simulink library "AtomicLibrary"
PostLoadFcn:
  | PacketBusGenerator; RailCabBusGenerator
(part 6 of 8)

== matlab function UserInterface/Link Layer HMI_STRATEGYREQUEST.provider/Receive Packet ==
  data: packetFrom input; packetMsg input; packetParam input; eventQueueIn input uint8; eventParamQueueIn input double; eventQueue output uint8; eventParamQueue output double; bufferOverflow output boolean
function [eventQueue, eventParamQueue, bufferOverflow] = receivePacket(packetFrom, packetMsg, packetParam, eventQueueIn, eventParamQueueIn)
%#eml
% This function receives packets and adds them to the event queue.
% A packet consists of a source, a message and an optional parameter for 
% the message. Source and message are contained at position 1 and 2 in the 
% eventQueue. Because of the different data type the parameter has his own 
% queue eventParamQueue.

%Constants
SOURCE = 2;
MESSAGE = 1;
BUS_SIZE = numel(packetFrom);
QUEUE_SIZE = 10;

%Init
eventQueue = eventQueueIn;
eventParamQueue = eventParamQueueIn;
bufferOverflow = false;

%New incoming packet
for i = 1:BUS_SIZE
    if packetFrom(i) ~= 0 
        bufferOverflow = true;
        %Add it to the incoming event Queue
        for j = 1:QUEUE_SIZE
            %Search for an empty place
            if eventQueue(j,SOURCE) == 0
                eventQueue(j,SOURCE)    = packetFrom(i);
                eventQueue(j,MESSAGE)   = packetMsg(i);
                eventParamQueue(j)      = packetParam(i);
                bufferOverflow = false;
                break;
            end
        end        
    else
        break;
    end
end

== matlab function UserInterface/Link Layer HMI_STRATEGYREQUEST.provider/Send Packet ==
  data: busSizeSignal input; eventQueueIn input uint8; eventParamQueueIn input double; packetMsg output; packetParam output; eventQueue output uint8; eventParamQueue output double
function [packetMsg, packetParam, eventQueue, eventParamQueue] = sendPacket(busSizeSignal, eventQueueIn, eventParamQueueIn)
%#eml

% This function creates packets from the event queue. A packet consists
% of a destination, a message and an optional parameter for the message.
% Destination and message are contained at position 1 and 2 in the 
% eventQueue. Because of the different data type the parameter has his own 
% queue eventParamQueue.

%Constants
DESTINATION = 2;
MESSAGE = 1;
QUEUE_SIZE = 10;

busSize = numel(busSizeSignal);

%Init
eventQueue = eventQueueIn;
eventParamQueue = eventParamQueueIn;
packetMsg = zeros(1,busSize,'uint16');
packetParam = zeros(1,busSize,'double');

%There is an event in the queue
for i = 1:busSize   
    if eventQueue(1,DESTINATION) ~= 0 || eventQueue(1,MESSAGE) ~= 0
        %Create packet from the firs entry in the queue
        packetMsg(i)   = uint16(eventQueue(1,MESSAGE));
        packetParam(i) = eventParamQueue(1);
        %Remove the event from the queue
        for j=1:QUEUE_SIZE - 1
            eventQueue(j,DESTINATION)   = eventQueue(j+1,DESTINATION);
            eventQueue(j,MESSAGE)       = eventQueue(j+1,MESSAGE);
            eventParamQueue(j)          = eventParamQueue(j+1);
        end
        %Set last element to zero
        eventQueue(QUEUE_SIZE,DESTINATION)  = 0;
        eventQueue(QUEUE_SIZE,MESSAGE)      = 0;
        eventParamQueue(QUEUE_SIZE)    = 0;
    else
        break;
    end
end

== matlab function UserInterface/Link Layer HMI_RESET.master/DataLinkLayer/Embedded MATLAB Function ==
  data: snd_from_in input; snd_to_in input; snd_msg_in input; snd_param_in input; recv_from_in input; recv_to_in input; recv_msg_in input; recv_param_in input; recv_pkgid_in input uint32; recv_time_in input; currentTime input; from output; to output; msg output; param output; pkgid output; recv_from_out output; recv_msg_out output; recv_param_out output; time output; queue_sending_ratio output; queue_received_ratio output; queue_ack_ratio output
function [from, to, msg, param, pkgid, recv_from_out, recv_msg_out, recv_param_out, time, queue_sending_ratio, queue_received_ratio, queue_ack_ratio] = ackHandler(snd_from_in, snd_to_in, snd_msg_in, snd_param_in, recv_from_in, recv_to_in, recv_msg_in, recv_param_in, recv_pkgid_in, recv_time_in, currentTime)
%#eml
eml.extrinsic('warning', 'disp', 'fprintf');

%Constants
BUS_SIZE =  numel(snd_msg_in);
TIMEOUT_ACK     = 2.0;
MSG_ACK         = 255;
QUEUE_SIZE_SENDING = 10 * BUS_SIZE;
QUEUE_SIZE_ACK  = 10* BUS_SIZE;
QUEUE_SIZE_RECEIVED = 10 *BUS_SIZE;


%Init
from    = zeros(1,BUS_SIZE,'uint8');
to      = zeros(1,BUS_SIZE,'uint8');
msg     = zeros(1,BUS_SIZE,'uint16');
param   = zeros(1,BUS_SIZE,'double');
pkgid   = zeros(1,BUS_SIZE,'uint32');
time    = zeros(1,BUS_SIZE,'double');
 
recv_from_out    = zeros(1,BUS_SIZE,'uint8');
recv_msg_out     = zeros(1,BUS_SIZE,'uint16');
recv_param_out   = zeros(1,BUS_SIZE,'double');


recv_in = bus(recv_from_in, recv_to_in, recv_msg_in, recv_param_in, recv_pkgid_in, recv_time_in, BUS_SIZE);



%Persistent variables
persistent sendingQueue ackQueue receivedQueue lastPkgid

if isempty(lastPkgid)
    lastPkgid = uint32(0);
end

if isempty(sendingQueue)
    sendingQueue = repmat(packet(0,0,0,0,0,0), 1, QUEUE_SIZE_SENDING);
end

if isempty(ackQueue)
    ackQueue = repmat(packet(0,0,0,0,0,0), 1, QUEUE_SIZE_ACK);
end

if isempty(receivedQueue)
    receivedQueue = repmat(packet(0, 0, 0, 0, 0, 0), 1, QUEUE_SIZE_RECEIVED);
end

%compute stats
queue_sending_ratio = queueNumElements(sendingQueue)/QUEUE_SIZE_SENDING;
queue_ack_ratio = queueNumElements(ackQueue)/QUEUE_SIZE_ACK;
queue_received_ratio = queueNumElements(receivedQueue)/QUEUE_SIZE_RECEIVED;

%Step 1: Check for a new outgoing packet
for i = 1:BUS_SIZE    
    if snd_msg_in(i) ~= 0
        lastPkgid = lastPkgid +1;
        outgoing = packet(snd_from_in, snd_to_in, snd_msg_in(i), snd_param_in(i), lastPkgid, currentTime);

        %Add packet so the outgoing queue
        sendingQueue = enqueue(sendingQueue, outgoing); 
    end
end
    
%Step 2: Check for a new incoming packet
for i = 1:length(recv_in)
    incoming = packet(recv_in(i).from, recv_in(i).to, recv_in(i).msg, recv_in(i).param, recv_in(i).pkgid, recv_in(i).time);
    if incoming.from ~= 0 && incoming.to == snd_from_in
        if incoming.msg == MSG_ACK
            %Remove packet from ackQueue
            for j=1:length(ackQueue)
                if ackQueue(j).pkgid == uint32(incoming.param)
                    ackQueue = dequeue(ackQueue,j);
                    break;
                end
            end
        else
            %Send ACK
            ackPacket = packet(incoming.to, incoming.from, MSG_ACK, double(incoming.pkgid),incoming.pkgid, currentTime);
            sendingQueue = enqueue(sendingQueue,ackPacket);

            %Check for duplicated packets
            duplicatedPacket = false;
            for j=1:length(receivedQueue)
                if receivedQueue(j).pkgid == incoming.pkgid && receivedQueue(j).from == incoming.from
                    duplicatedPacket = true;
                    break;
                end
            end

            if duplicatedPacket == false
                %save packet
                receivedQueue = enqueue(receivedQueue, incoming);            
            end
        end
    end
end

%Step 3: Forward incoming packet
for i = 1:BUS_SIZE
    if receivedQueue(1).from ~= 0
        recv_from_out(i)    = receivedQueue(1).from;
        recv_msg_out(i)     = receivedQueue(1).msg;
        recv_param_out(i)   = receivedQueue(1).param;
        receivedQueue = dequeue(receivedQueue,1);
    else
        break;
    end
end

%Step 4: Timeout reached? Send packet again
for i = 1:length(ackQueue)
    if ackQueue(i).to ~= 0
        if ackQueue(i).time + TIMEOUT_ACK <= currentTime
            %Reset counter
            ackQueue(i).time = currentTime;
            %Send again
            sendingQueue = enqueue(sendingQueue, ackQueue(i));
            %Remove packet from ackQueue
            ackQueue = dequeue(ackQueue, i);
        end
    end
end


%Step 5: Send outgoing packet
for i = 1:BUS_SIZE
    if sendingQueue(1).to ~= 0    
        from(i)    = sendingQueue(1).from;
        to(i)      = sendingQueue(1).to;
        msg(i)     = sendingQueue(1).msg;
        param(i)   = sendingQueue(1).param;
        pkgid(i)   = sendingQueue(1).pkgid;
        time(i)    = sendingQueue(1).time;

        %Add it to the ack queue
        if sendingQueue(1).msg ~= MSG_ACK
            ackQueue = enqueue(ackQueue, sendingQueue(1));
        end

        %remove packet from sending queue
        sendingQueue = dequeue(sendingQueue, 1);    
    else
        break;
    end
end


%%%%%%%%%%%%%%%%%%%%%%%%%%%%%%%%%%%%%%%%%%%%%%%%%%%%%%%%%%%%%%%%%%%%%%%%%%%
%%                          H E L P E R
%%%%%%%%%%%%%%%%%%%%%%%%%%%%%%%%%%%%%%%%%%%%%%%%%%%%%%%%%%%%%%%%%%%%%%%%%%%

function p = packet(from, to, msg, param, pkgid, time)
%#eml
%Defines a packet
p = struct('from', uint8(from),'to', uint8(to),'msg', uint16(msg),'param', double(param),'pkgid', uint32(pkgid), 'time', double(time));

function bus = bus(from, to, msg, param, pkgid, time, size) %emp
%Create an empty bus
bus = repmat(packet(0,0,0,0,0,0), 1, size);
for i=1:size
    bus(i) = packet(from(i), to(i), msg(i), param(i), pkgid(i), time(i));
end


function queue = enqueue(queue, packet)
%#eml
eml.extrinsic('warning', 'sprintf');
for i = 1:length(queue)
    if queue(i).to == 0
        queue(i) = packet;
        return;
    end
end
warning('RailCab:DataLinkLayer', 'DataLinkLayer Buffer overflow. Dropping packet  %3u: %u->%u :%3u (%.1f) @%.2f', packet.pkgid, packet.from, packet.to, packet.msg, packet.param, packet.time);

function queue = dequeue(queue, index)
%#eml
assert(index <= length(queue))
for i=index:length(queue)-1;
    queue(i) = queue(i+1);
end
queue(length(queue)) = packet(0,0,0,0,0,0);

function num = queueNumElements(queue)
%#eml
num = 0;
for i = 1:length(queue)
    if queue(i).to ~= uint8(0)
        num = num+1;
    end
end    

function packetString = toString(packet) %#eml
eml.extrinsic('sprintf');
packetString = sprintf('%3u: %u->%u :%3u (%.1f) @%.2f', packet.pkgid, packet.from, packet.to, packet.msg, packet.param, packet.time);

== matlab function UserInterface/Link Layer HMI_RESET.master/Receive Packet ==
  data: packetFrom input; packetMsg input; packetParam input; eventQueueIn input uint8; eventParamQueueIn input double; eventQueue output uint8; eventParamQueue output double; bufferOverflow output boolean
function [eventQueue, eventParamQueue, bufferOverflow] = receivePacket(packetFrom, packetMsg, packetParam, eventQueueIn, eventParamQueueIn)
%#eml
% This function receives packets and adds them to the event queue.
% A packet consists of a source, a message and an optional parameter for 
% the message. Source and message are contained at position 1 and 2 in the 
% eventQueue. Because of the different data type the parameter has his own 
% queue eventParamQueue.

%Constants
SOURCE = 2;
MESSAGE = 1;
BUS_SIZE = numel(packetFrom);
QUEUE_SIZE = 10;

%Init
eventQueue = eventQueueIn;
eventParamQueue = eventParamQueueIn;
bufferOverflow = false;

%New incoming packet
for i = 1:BUS_SIZE
    if packetFrom(i) ~= 0 
        bufferOverflow = true;
        %Add it to the incoming event Queue
        for j = 1:QUEUE_SIZE
            %Search for an empty place
            if eventQueue(j,SOURCE) == 0
                eventQueue(j,SOURCE)    = packetFrom(i);
                eventQueue(j,MESSAGE)   = packetMsg(i);
                eventParamQueue(j)      = packetParam(i);
                bufferOverflow = false;
                break;
            end
        end        
    else
        break;
    end
end

== matlab function UserInterface/Link Layer HMI_RESET.master/Send Packet ==
  data: busSizeSignal input; eventQueueIn input uint8; eventParamQueueIn input double; packetMsg output; packetParam output; eventQueue output uint8; eventParamQueue output double
function [packetMsg, packetParam, eventQueue, eventParamQueue] = sendPacket(busSizeSignal, eventQueueIn, eventParamQueueIn)
%#eml

% This function creates packets from the event queue. A packet consists
% of a destination, a message and an optional parameter for the message.
% Destination and message are contained at position 1 and 2 in the 
% eventQueue. Because of the different data type the parameter has his own 
% queue eventParamQueue.

%Constants
DESTINATION = 2;
MESSAGE = 1;
QUEUE_SIZE = 10;

busSize = numel(busSizeSignal);

%Init
eventQueue = eventQueueIn;
eventParamQueue = eventParamQueueIn;
packetMsg = zeros(1,busSize,'uint16');
packetParam = zeros(1,busSize,'double');

%There is an event in the queue
for i = 1:busSize   
    if eventQueue(1,DESTINATION) ~= 0 || eventQueue(1,MESSAGE) ~= 0
        %Create packet from the firs entry in the queue
        packetMsg(i)   = uint16(eventQueue(1,MESSAGE));
        packetParam(i) = eventParamQueue(1);
        %Remove the event from the queue
        for j=1:QUEUE_SIZE - 1
            eventQueue(j,DESTINATION)   = eventQueue(j+1,DESTINATION);
            eventQueue(j,MESSAGE)       = eventQueue(j+1,MESSAGE);
            eventParamQueue(j)          = eventParamQueue(j+1);
        end
        %Set last element to zero
        eventQueue(QUEUE_SIZE,DESTINATION)  = 0;
        eventQueue(QUEUE_SIZE,MESSAGE)      = 0;
        eventParamQueue(QUEUE_SIZE)    = 0;
    else
        break;
    end
end

== matlab function UserInterface/Link Layer HMI_STRATEGY.master/DataLinkLayer/Embedded MATLAB Function ==
  data: snd_from_in input; snd_to_in input; snd_msg_in input; snd_param_in input; recv_from_in input; recv_to_in input; recv_msg_in input; recv_param_in input; recv_pkgid_in input uint32; recv_time_in input; currentTime input; from output; to output; msg output; param output; pkgid output; recv_from_out output; recv_msg_out output; recv_param_out output; time output; queue_sending_ratio output; queue_received_ratio output; queue_ack_ratio output
function [from, to, msg, param, pkgid, recv_from_out, recv_msg_out, recv_param_out, time, queue_sending_ratio, queue_received_ratio, queue_ack_ratio] = ackHandler(snd_from_in, snd_to_in, snd_msg_in, snd_param_in, recv_from_in, recv_to_in, recv_msg_in, recv_param_in, recv_pkgid_in, recv_time_in, currentTime)
%#eml
eml.extrinsic('warning', 'disp', 'fprintf');

%Constants
BUS_SIZE =  numel(snd_msg_in);
TIMEOUT_ACK     = 2.0;
MSG_ACK         = 255;
QUEUE_SIZE_SENDING = 10 * BUS_SIZE;
QUEUE_SIZE_ACK  = 10* BUS_SIZE;
QUEUE_SIZE_RECEIVED = 10 *BUS_SIZE;


%Init
from    = zeros(1,BUS_SIZE,'uint8');
to      = zeros(1,BUS_SIZE,'uint8');
msg     = zeros(1,BUS_SIZE,'uint16');
param   = zeros(1,BUS_SIZE,'double');
pkgid   = zeros(1,BUS_SIZE,'uint32');
time    = zeros(1,BUS_SIZE,'double');
 
recv_from_out    = zeros(1,BUS_SIZE,'uint8');
recv_msg_out     = zeros(1,BUS_SIZE,'uint16');
recv_param_out   = zeros(1,BUS_SIZE,'double');


recv_in = bus(recv_from_in, recv_to_in, recv_msg_in, recv_param_in, recv_pkgid_in, recv_time_in, BUS_SIZE);



%Persistent variables
persistent sendingQueue ackQueue receivedQueue lastPkgid

if isempty(lastPkgid)
    lastPkgid = uint32(0);
end

if isempty(sendingQueue)
    sendingQueue = repmat(packet(0,0,0,0,0,0), 1, QUEUE_SIZE_SENDING);
end

if isempty(ackQueue)
    ackQueue = repmat(packet(0,0,0,0,0,0), 1, QUEUE_SIZE_ACK);
end

if isempty(receivedQueue)
    receivedQueue = repmat(packet(0, 0, 0, 0, 0, 0), 1, QUEUE_SIZE_RECEIVED);
end

%compute stats
queue_sending_ratio = queueNumElements(sendingQueue)/QUEUE_SIZE_SENDING;
queue_ack_ratio = queueNumElements(ackQueue)/QUEUE_SIZE_ACK;
queue_received_ratio = queueNumElements(receivedQueue)/QUEUE_SIZE_RECEIVED;

%Step 1: Check for a new outgoing packet
for i = 1:BUS_SIZE    
    if snd_msg_in(i) ~= 0
        lastPkgid = lastPkgid +1;
        outgoing = packet(snd_from_in, snd_to_in, snd_msg_in(i), snd_param_in(i), lastPkgid, currentTime);

        %Add packet so the outgoing queue
        sendingQueue = enqueue(sendingQueue, outgoing); 
    end
end
    
%Step 2: Check for a new incoming packet
for i = 1:length(recv_in)
    incoming = packet(recv_in(i).from, recv_in(i).to, recv_in(i).msg, recv_in(i).param, recv_in(i).pkgid, recv_in(i).time);
    if incoming.from ~= 0 && incoming.to == snd_from_in
        if incoming.msg == MSG_ACK
            %Remove packet from ackQueue
            for j=1:length(ackQueue)
                if ackQueue(j).pkgid == uint32(incoming.param)
                    ackQueue = dequeue(ackQueue,j);
                    break;
                end
            end
        else
            %Send ACK
            ackPacket = packet(incoming.to, incoming.from, MSG_ACK, double(incoming.pkgid),incoming.pkgid, currentTime);
            sendingQueue = enqueue(sendingQueue,ackPacket);

            %Check for duplicated packets
            duplicatedPacket = false;
            for j=1:length(receivedQueue)
                if receivedQueue(j).pkgid == incoming.pkgid && receivedQueue(j).from == incoming.from
                    duplicatedPacket = true;
                    break;
                end
            end

            if duplicatedPacket == false
                %save packet
                receivedQueue = enqueue(receivedQueue, incoming);            
            end
        end
    end
end

%Step 3: Forward incoming packet
for i = 1:BUS_SIZE
    if receivedQueue(1).from ~= 0
        recv_from_out(i)    = receivedQueue(1).from;
        recv_msg_out(i)     = receivedQueue(1).msg;
        recv_param_out(i)   = receivedQueue(1).param;
        receivedQueue = dequeue(receivedQueue,1);
    else
        break;
    end
end

%Step 4: Timeout reached? Send packet again
for i = 1:length(ackQueue)
    if ackQueue(i).to ~= 0
        if ackQueue(i).time + TIMEOUT_ACK <= currentTime
            %Reset counter
            ackQueue(i).time = currentTime;
            %Send again
            sendingQueue = enqueue(sendingQueue, ackQueue(i));
            %Remove packet from ackQueue
            ackQueue = dequeue(ackQueue, i);
        end
    end
end


%Step 5: Send outgoing packet
for i = 1:BUS_SIZE
    if sendingQueue(1).to ~= 0    
        from(i)    = sendingQueue(1).from;
        to(i)      = sendingQueue(1).to;
        msg(i)     = sendingQueue(1).msg;
        param(i)   = sendingQueue(1).param;
        pkgid(i)   = sendingQueue(1).pkgid;
        time(i)    = sendingQueue(1).time;

        %Add it to the ack queue
        if sendingQueue(1).msg ~= MSG_ACK
            ackQueue = enqueue(ackQueue, sendingQueue(1));
        end

        %remove packet from sending queue
        sendingQueue = dequeue(sendingQueue, 1);    
    else
        break;
    end
end


%%%%%%%%%%%%%%%%%%%%%%%%%%%%%%%%%%%%%%%%%%%%%%%%%%%%%%%%%%%%%%%%%%%%%%%%%%%
%%                          H E L P E R
%%%%%%%%%%%%%%%%%%%%%%%%%%%%%%%%%%%%%%%%%%%%%%%%%%%%%%%%%%%%%%%%%%%%%%%%%%%

function p = packet(from, to, msg, param, pkgid, time)
%#eml
%Defines a packet
p = struct('from', uint8(from),'to', uint8(to),'msg', uint16(msg),'param', double(param),'pkgid', uint32(pkgid), 'time', double(time));

function bus = bus(from, to, msg, param, pkgid, time, size) %emp
%Create an empty bus
bus = repmat(packet(0,0,0,0,0,0), 1, size);
for i=1:size
    bus(i) = packet(from(i), to(i), msg(i), param(i), pkgid(i), time(i));
end


function queue = enqueue(queue, packet)
%#eml
eml.extrinsic('warning', 'sprintf');
for i = 1:length(queue)
    if queue(i).to == 0
        queue(i) = packet;
        return;
    end
end
warning('RailCab:DataLinkLayer', 'DataLinkLayer Buffer overflow. Dropping packet  %3u: %u->%u :%3u (%.1f) @%.2f', packet.pkgid, packet.from, packet.to, packet.msg, packet.param, packet.time);

function queue = dequeue(queue, index)
%#eml
assert(index <= length(queue))
for i=index:length(queue)-1;
    queue(i) = queue(i+1);
end
queue(length(queue)) = packet(0,0,0,0,0,0);

function num = queueNumElements(queue)
%#eml
num = 0;
for i = 1:length(queue)
    if queue(i).to ~= uint8(0)
        num = num+1;
    end
end    

function packetString = toString(packet) %#eml
eml.extrinsic('sprintf');
packetString = sprintf('%3u: %u->%u :%3u (%.1f) @%.2f', packet.pkgid, packet.from, packet.to, packet.msg, packet.param, packet.time);

== matlab function UserInterface/Link Layer HMI_STRATEGY.master/Receive Packet ==
  data: packetFrom input; packetMsg input; packetParam input; eventQueueIn input uint8; eventParamQueueIn input double; eventQueue output uint8; eventParamQueue output double; bufferOverflow output boolean
function [eventQueue, eventParamQueue, bufferOverflow] = receivePacket(packetFrom, packetMsg, packetParam, eventQueueIn, eventParamQueueIn)
%#eml
% This function receives packets and adds them to the event queue.
% A packet consists of a source, a message and an optional parameter for 
% the message. Source and message are contained at position 1 and 2 in the 
% eventQueue. Because of the different data type the parameter has his own 
% queue eventParamQueue.

%Constants
SOURCE = 2;
MESSAGE = 1;
BUS_SIZE = numel(packetFrom);
QUEUE_SIZE = 10;

%Init
eventQueue = eventQueueIn;
eventParamQueue = eventParamQueueIn;
bufferOverflow = false;

%New incoming packet
for i = 1:BUS_SIZE
    if packetFrom(i) ~= 0 
        bufferOverflow = true;
        %Add it to the incoming event Queue
        for j = 1:QUEUE_SIZE
            %Search for an empty place
            if eventQueue(j,SOURCE) == 0
                eventQueue(j,SOURCE)    = packetFrom(i);
                eventQueue(j,MESSAGE)   = packetMsg(i);
                eventParamQueue(j)      = packetParam(i);
                bufferOverflow = false;
                break;
            end
        end        
    else
        break;
    end
end

== matlab function UserInterface/Link Layer HMI_STRATEGY.master/Send Packet ==
  data: busSizeSignal input; eventQueueIn input uint8; eventParamQueueIn input double; packetMsg output; packetParam output; eventQueue output uint8; eventParamQueue output double
function [packetMsg, packetParam, eventQueue, eventParamQueue] = sendPacket(busSizeSignal, eventQueueIn, eventParamQueueIn)
%#eml

% This function creates packets from the event queue. A packet consists
% of a destination, a message and an optional parameter for the message.
% Destination and message are contained at position 1 and 2 in the 
% eventQueue. Because of the different data type the parameter has his own 
% queue eventParamQueue.

%Constants
DESTINATION = 2;
MESSAGE = 1;
QUEUE_SIZE = 10;

busSize = numel(busSizeSignal);

%Init
eventQueue = eventQueueIn;
eventParamQueue = eventParamQueueIn;
packetMsg = zeros(1,busSize,'uint16');
packetParam = zeros(1,busSize,'double');

%There is an event in the queue
for i = 1:busSize   
    if eventQueue(1,DESTINATION) ~= 0 || eventQueue(1,MESSAGE) ~= 0
        %Create packet from the firs entry in the queue
        packetMsg(i)   = uint16(eventQueue(1,MESSAGE));
        packetParam(i) = eventParamQueue(1);
        %Remove the event from the queue
        for j=1:QUEUE_SIZE - 1
            eventQueue(j,DESTINATION)   = eventQueue(j+1,DESTINATION);
            eventQueue(j,MESSAGE)       = eventQueue(j+1,MESSAGE);
            eventParamQueue(j)          = eventParamQueue(j+1);
        end
        %Set last element to zero
        eventQueue(QUEUE_SIZE,DESTINATION)  = 0;
        eventQueue(QUEUE_SIZE,MESSAGE)      = 0;
        eventParamQueue(QUEUE_SIZE)    = 0;
    else
        break;
    end
end

== matlab function UserInterface/Link Layer STATUS.slave/DataLinkLayer/Embedded MATLAB Function ==
  data: snd_from_in input; snd_to_in input; snd_msg_in input; snd_param_in input; recv_from_in input; recv_to_in input; recv_msg_in input; recv_param_in input; recv_pkgid_in input uint32; recv_time_in input; currentTime input; from output; to output; msg output; param output; pkgid output; recv_from_out output; recv_msg_out output; recv_param_out output; time output; queue_sending_ratio output; queue_received_ratio output; queue_ack_ratio output
function [from, to, msg, param, pkgid, recv_from_out, recv_msg_out, recv_param_out, time, queue_sending_ratio, queue_received_ratio, queue_ack_ratio] = ackHandler(snd_from_in, snd_to_in, snd_msg_in, snd_param_in, recv_from_in, recv_to_in, recv_msg_in, recv_param_in, recv_pkgid_in, recv_time_in, currentTime)
%#eml
eml.extrinsic('warning', 'disp', 'fprintf');

%Constants
BUS_SIZE =  numel(snd_msg_in);
TIMEOUT_ACK     = 2.0;
MSG_ACK         = 255;
QUEUE_SIZE_SENDING = 10 * BUS_SIZE;
QUEUE_SIZE_ACK  = 10* BUS_SIZE;
QUEUE_SIZE_RECEIVED = 10 *BUS_SIZE;


%Init
from    = zeros(1,BUS_SIZE,'uint8');
to      = zeros(1,BUS_SIZE,'uint8');
msg     = zeros(1,BUS_SIZE,'uint16');
param   = zeros(1,BUS_SIZE,'double');
pkgid   = zeros(1,BUS_SIZE,'uint32');
time    = zeros(1,BUS_SIZE,'double');
 
recv_from_out    = zeros(1,BUS_SIZE,'uint8');
recv_msg_out     = zeros(1,BUS_SIZE,'uint16');
recv_param_out   = zeros(1,BUS_SIZE,'double');


recv_in = bus(recv_from_in, recv_to_in, recv_msg_in, recv_param_in, recv_pkgid_in, recv_time_in, BUS_SIZE);



%Persistent variables
persistent sendingQueue ackQueue receivedQueue lastPkgid

if isempty(lastPkgid)
    lastPkgid = uint32(0);
end

if isempty(sendingQueue)
    sendingQueue = repmat(packet(0,0,0,0,0,0), 1, QUEUE_SIZE_SENDING);
end

if isempty(ackQueue)
    ackQueue = repmat(packet(0,0,0,0,0,0), 1, QUEUE_SIZE_ACK);
end

if isempty(receivedQueue)
    receivedQueue = repmat(packet(0, 0, 0, 0, 0, 0), 1, QUEUE_SIZE_RECEIVED);
end

%compute stats
queue_sending_ratio = queueNumElements(sendingQueue)/QUEUE_SIZE_SENDING;
queue_ack_ratio = queueNumElements(ackQueue)/QUEUE_SIZE_ACK;
queue_received_ratio = queueNumElements(receivedQueue)/QUEUE_SIZE_RECEIVED;

%Step 1: Check for a new outgoing packet
for i = 1:BUS_SIZE    
    if snd_msg_in(i) ~= 0
        lastPkgid = lastPkgid +1;
        outgoing = packet(snd_from_in, snd_to_in, snd_msg_in(i), snd_param_in(i), lastPkgid, currentTime);

        %Add packet so the outgoing queue
        sendingQueue = enqueue(sendingQueue, outgoing); 
    end
end
    
%Step 2: Check for a new incoming packet
for i = 1:length(recv_in)
    incoming = packet(recv_in(i).from, recv_in(i).to, recv_in(i).msg, recv_in(i).param, recv_in(i).pkgid, recv_in(i).time);
    if incoming.from ~= 0 && incoming.to == snd_from_in
        if incoming.msg == MSG_ACK
            %Remove packet from ackQueue
            for j=1:length(ackQueue)
                if ackQueue(j).pkgid == uint32(incoming.param)
                    ackQueue = dequeue(ackQueue,j);
                    break;
                end
            end
        else
            %Send ACK
            ackPacket = packet(incoming.to, incoming.from, MSG_ACK, double(incoming.pkgid),incoming.pkgid, currentTime);
            sendingQueue = enqueue(sendingQueue,ackPacket);

            %Check for duplicated packets
            duplicatedPacket = false;
            for j=1:length(receivedQueue)
                if receivedQueue(j).pkgid == incoming.pkgid && receivedQueue(j).from == incoming.from
                    duplicatedPacket = true;
                    break;
                end
            end

            if duplicatedPacket == false
                %save packet
                receivedQueue = enqueue(receivedQueue, incoming);            
            end
        end
    end
end

%Step 3: Forward incoming packet
for i = 1:BUS_SIZE
    if receivedQueue(1).from ~= 0
        recv_from_out(i)    = receivedQueue(1).from;
        recv_msg_out(i)     = receivedQueue(1).msg;
        recv_param_out(i)   = receivedQueue(1).param;
        receivedQueue = dequeue(receivedQueue,1);
    else
        break;
    end
end

%Step 4: Timeout reached? Send packet again
for i = 1:length(ackQueue)
    if ackQueue(i).to ~= 0
        if ackQueue(i).time + TIMEOUT_ACK <= currentTime
            %Reset counter
            ackQueue(i).time = currentTime;
            %Send again
            sendingQueue = enqueue(sendingQueue, ackQueue(i));
            %Remove packet from ackQueue
            ackQueue = dequeue(ackQueue, i);
        end
    end
end


%Step 5: Send outgoing packet
for i = 1:BUS_SIZE
    if sendingQueue(1).to ~= 0    
        from(i)    = sendingQueue(1).from;
        to(i)      = sendingQueue(1).to;
        msg(i)     = sendingQueue(1).msg;
        param(i)   = sendingQueue(1).param;
        pkgid(i)   = sendingQueue(1).pkgid;
        time(i)    = sendingQueue(1).time;

        %Add it to the ack queue
        if sendingQueue(1).msg ~= MSG_ACK
            ackQueue = enqueue(ackQueue, sendingQueue(1));
        end

        %remove packet from sending queue
        sendingQueue = dequeue(sendingQueue, 1);    
    else
        break;
    end
end


%%%%%%%%%%%%%%%%%%%%%%%%%%%%%%%%%%%%%%%%%%%%%%%%%%%%%%%%%%%%%%%%%%%%%%%%%%%
%%                          H E L P E R
%%%%%%%%%%%%%%%%%%%%%%%%%%%%%%%%%%%%%%%%%%%%%%%%%%%%%%%%%%%%%%%%%%%%%%%%%%%

function p = packet(from, to, msg, param, pkgid, time)
%#eml
%Defines a packet
p = struct('from', uint8(from),'to', uint8(to),'msg', uint16(msg),'param', double(param),'pkgid', uint32(pkgid), 'time', double(time));

function bus = bus(from, to, msg, param, pkgid, time, size) %emp
%Create an empty bus
bus = repmat(packet(0,0,0,0,0,0), 1, size);
for i=1:size
    bus(i) = packet(from(i), to(i), msg(i), param(i), pkgid(i), time(i));
end


function queue = enqueue(queue, packet)
%#eml
eml.extrinsic('warning', 'sprintf');
for i = 1:length(queue)
    if queue(i).to == 0
        queue(i) = packet;
        return;
    end
end
warning('RailCab:DataLinkLayer', 'DataLinkLayer Buffer overflow. Dropping packet  %3u: %u->%u :%3u (%.1f) @%.2f', packet.pkgid, packet.from, packet.to, packet.msg, packet.param, packet.time);

function queue = dequeue(queue, index)
%#eml
assert(index <= length(queue))
for i=index:length(queue)-1;
    queue(i) = queue(i+1);
end
queue(length(queue)) = packet(0,0,0,0,0,0);

function num = queueNumElements(queue)
%#eml
num = 0;
for i = 1:length(queue)
    if queue(i).to ~= uint8(0)
        num = num+1;
    end
end    

function packetString = toString(packet) %#eml
eml.extrinsic('sprintf');
packetString = sprintf('%3u: %u->%u :%3u (%.1f) @%.2f', packet.pkgid, packet.from, packet.to, packet.msg, packet.param, packet.time);

== matlab function UserInterface/Link Layer STATUS.slave/Receive Packet ==
  data: packetFrom input; packetMsg input; packetParam input; eventQueueIn input uint8; eventParamQueueIn input double; eventQueue output uint8; eventParamQueue output double; bufferOverflow output boolean
function [eventQueue, eventParamQueue, bufferOverflow] = receivePacket(packetFrom, packetMsg, packetParam, eventQueueIn, eventParamQueueIn)
%#eml
% This function receives packets and adds them to the event queue.
% A packet consists of a source, a message and an optional parameter for 
% the message. Source and message are contained at position 1 and 2 in the 
% eventQueue. Because of the different data type the parameter has his own 
% queue eventParamQueue.

%Constants
SOURCE = 2;
MESSAGE = 1;
BUS_SIZE = numel(packetFrom);
QUEUE_SIZE = 10;

%Init
eventQueue = eventQueueIn;
eventParamQueue = eventParamQueueIn;
bufferOverflow = false;

%New incoming packet
for i = 1:BUS_SIZE
    if packetFrom(i) ~= 0 
        bufferOverflow = true;
        %Add it to the incoming event Queue
        for j = 1:QUEUE_SIZE
            %Search for an empty place
            if eventQueue(j,SOURCE) == 0
                eventQueue(j,SOURCE)    = packetFrom(i);
                eventQueue(j,MESSAGE)   = packetMsg(i);
                eventParamQueue(j)      = packetParam(i);
                bufferOverflow = false;
                break;
            end
        end        
    else
        break;
    end
end

== matlab function UserInterface/Link Layer STATUS.slave/Send Packet ==
  data: busSizeSignal input; eventQueueIn input uint8; eventParamQueueIn input double; packetMsg output; packetParam output; eventQueue output uint8; eventParamQueue output double
function [packetMsg, packetParam, eventQueue, eventParamQueue] = sendPacket(busSizeSignal, eventQueueIn, eventParamQueueIn)
%#eml

% This function creates packets from the event queue. A packet consists
% of a destination, a message and an optional parameter for the message.
% Destination and message are contained at position 1 and 2 in the 
% eventQueue. Because of the different data type the parameter has his own 
% queue eventParamQueue.

%Constants
DESTINATION = 2;
MESSAGE = 1;
QUEUE_SIZE = 10;

busSize = numel(busSizeSignal);

%Init
eventQueue = eventQueueIn;
eventParamQueue = eventParamQueueIn;
packetMsg = zeros(1,busSize,'uint16');
packetParam = zeros(1,busSize,'double');

%There is an event in the queue
for i = 1:busSize   
    if eventQueue(1,DESTINATION) ~= 0 || eventQueue(1,MESSAGE) ~= 0
        %Create packet from the firs entry in the queue
        packetMsg(i)   = uint16(eventQueue(1,MESSAGE));
        packetParam(i) = eventParamQueue(1);
        %Remove the event from the queue
        for j=1:QUEUE_SIZE - 1
            eventQueue(j,DESTINATION)   = eventQueue(j+1,DESTINATION);
            eventQueue(j,MESSAGE)       = eventQueue(j+1,MESSAGE);
            eventParamQueue(j)          = eventParamQueue(j+1);
        end
        %Set last element to zero
        eventQueue(QUEUE_SIZE,DESTINATION)  = 0;
        eventQueue(QUEUE_SIZE,MESSAGE)      = 0;
        eventParamQueue(QUEUE_SIZE)    = 0;
    else
        break;
    end
end

== matlab function UserInterface/Link Layer HMI_END.master/DataLinkLayer/Embedded MATLAB Function ==
  data: snd_from_in input; snd_to_in input; snd_msg_in input; snd_param_in input; recv_from_in input; recv_to_in input; recv_msg_in input; recv_param_in input; recv_pkgid_in input uint32; recv_time_in input; currentTime input; from output; to output; msg output; param output; pkgid output; recv_from_out output; recv_msg_out output; recv_param_out output; time output; queue_sending_ratio output; queue_received_ratio output; queue_ack_ratio output
function [from, to, msg, param, pkgid, recv_from_out, recv_msg_out, recv_param_out, time, queue_sending_ratio, queue_received_ratio, queue_ack_ratio] = ackHandler(snd_from_in, snd_to_in, snd_msg_in, snd_param_in, recv_from_in, recv_to_in, recv_msg_in, recv_param_in, recv_pkgid_in, recv_time_in, currentTime)
%#eml
eml.extrinsic('warning', 'disp', 'fprintf');

%Constants
BUS_SIZE =  numel(snd_msg_in);
TIMEOUT_ACK     = 2.0;
MSG_ACK         = 255;
QUEUE_SIZE_SENDING = 10 * BUS_SIZE;
QUEUE_SIZE_ACK  = 10* BUS_SIZE;
QUEUE_SIZE_RECEIVED = 10 *BUS_SIZE;


%Init
from    = zeros(1,BUS_SIZE,'uint8');
to      = zeros(1,BUS_SIZE,'uint8');
msg     = zeros(1,BUS_SIZE,'uint16');
param   = zeros(1,BUS_SIZE,'double');
pkgid   = zeros(1,BUS_SIZE,'uint32');
time    = zeros(1,BUS_SIZE,'double');
 
recv_from_out    = zeros(1,BUS_SIZE,'uint8');
recv_msg_out     = zeros(1,BUS_SIZE,'uint16');
recv_param_out   = zeros(1,BUS_SIZE,'double');


recv_in = bus(recv_from_in, recv_to_in, recv_msg_in, recv_param_in, recv_pkgid_in, recv_time_in, BUS_SIZE);



%Persistent variables
persistent sendingQueue ackQueue receivedQueue lastPkgid

if isempty(lastPkgid)
    lastPkgid = uint32(0);
end

if isempty(sendingQueue)
    sendingQueue = repmat(packet(0,0,0,0,0,0), 1, QUEUE_SIZE_SENDING);
end

if isempty(ackQueue)
    ackQueue = repmat(packet(0,0,0,0,0,0), 1, QUEUE_SIZE_ACK);
end

if isempty(receivedQueue)
    receivedQueue = repmat(packet(0, 0, 0, 0, 0, 0), 1, QUEUE_SIZE_RECEIVED);
end

%compute stats
queue_sending_ratio = queueNumElements(sendingQueue)/QUEUE_SIZE_SENDING;
queue_ack_ratio = queueNumElements(ackQueue)/QUEUE_SIZE_ACK;
queue_received_ratio = queueNumElements(receivedQueue)/QUEUE_SIZE_RECEIVED;

%Step 1: Check for a new outgoing packet
for i = 1:BUS_SIZE    
    if snd_msg_in(i) ~= 0
        lastPkgid = lastPkgid +1;
        outgoing = packet(snd_from_in, snd_to_in, snd_msg_in(i), snd_param_in(i), lastPkgid, currentTime);

        %Add packet so the outgoing queue
        sendingQueue = enqueue(sendingQueue, outgoing); 
    end
end
    
%Step 2: Check for a new incoming packet
for i = 1:length(recv_in)
    incoming = packet(recv_in(i).from, recv_in(i).to, recv_in(i).msg, recv_in(i).param, recv_in(i).pkgid, recv_in(i).time);
    if incoming.from ~= 0 && incoming.to == snd_from_in
        if incoming.msg == MSG_ACK
            %Remove packet from ackQueue
            for j=1:length(ackQueue)
                if ackQueue(j).pkgid == uint32(incoming.param)
                    ackQueue = dequeue(ackQueue,j);
                    break;
                end
            end
        else
            %Send ACK
            ackPacket = packet(incoming.to, incoming.from, MSG_ACK, double(incoming.pkgid),incoming.pkgid, currentTime);
            sendingQueue = enqueue(sendingQueue,ackPacket);

            %Check for duplicated packets
            duplicatedPacket = false;
            for j=1:length(receivedQueue)
                if receivedQueue(j).pkgid == incoming.pkgid && receivedQueue(j).from == incoming.from
                    duplicatedPacket = true;
                    break;
                end
            end

            if duplicatedPacket == false
                %save packet
                receivedQueue = enqueue(receivedQueue, incoming);            
            end
        end
    end
end

%Step 3: Forward incoming packet
for i = 1:BUS_SIZE
    if receivedQueue(1).from ~= 0
        recv_from_out(i)    = receivedQueue(1).from;
        recv_msg_out(i)     = receivedQueue(1).msg;
        recv_param_out(i)   = receivedQueue(1).param;
        receivedQueue = dequeue(receivedQueue,1);
    else
        break;
    end
end

%Step 4: Timeout reached? Send packet again
for i = 1:length(ackQueue)
    if ackQueue(i).to ~= 0
        if ackQueue(i).time + TIMEOUT_ACK <= currentTime
            %Reset counter
            ackQueue(i).time = currentTime;
            %Send again
            sendingQueue = enqueue(sendingQueue, ackQueue(i));
            %Remove packet from ackQueue
            ackQueue = dequeue(ackQueue, i);
        end
    end
end


%Step 5: Send outgoing packet
for i = 1:BUS_SIZE
    if sendingQueue(1).to ~= 0    
        from(i)    = sendingQueue(1).from;
        to(i)      = sendingQueue(1).to;
        msg(i)     = sendingQueue(1).msg;
        param(i)   = sendingQueue(1).param;
        pkgid(i)   = sendingQueue(1).pkgid;
        time(i)    = sendingQueue(1).time;

        %Add it to the ack queue
        if sendingQueue(1).msg ~= MSG_ACK
            ackQueue = enqueue(ackQueue, sendingQueue(1));
        end

        %remove packet from sending queue
        sendingQueue = dequeue(sendingQueue, 1);    
    else
        break;
    end
end


%%%%%%%%%%%%%%%%%%%%%%%%%%%%%%%%%%%%%%%%%%%%%%%%%%%%%%%%%%%%%%%%%%%%%%%%%%%
%%                          H E L P E R
%%%%%%%%%%%%%%%%%%%%%%%%%%%%%%%%%%%%%%%%%%%%%%%%%%%%%%%%%%%%%%%%%%%%%%%%%%%

function p = packet(from, to, msg, param, pkgid, time)
%#eml
%Defines a packet
p = struct('from', uint8(from),'to', uint8(to),'msg', uint16(msg),'param', double(param),'pkgid', uint32(pkgid), 'time', double(time));

function bus = bus(from, to, msg, param, pkgid, time, size) %emp
%Create an empty bus
bus = repmat(packet(0,0,0,0,0,0), 1, size);
for i=1:size
    bus(i) = packet(from(i), to(i), msg(i), param(i), pkgid(i), time(i));
end


function queue = enqueue(queue, packet)
%#eml
eml.extrinsic('warning', 'sprintf');
for i = 1:length(queue)
    if queue(i).to == 0
        queue(i) = packet;
        return;
    end
end
warning('RailCab:DataLinkLayer', 'DataLinkLayer Buffer overflow. Dropping packet  %3u: %u->%u :%3u (%.1f) @%.2f', packet.pkgid, packet.from, packet.to, packet.msg, packet.param, packet.time);

function queue = dequeue(queue, index)
%#eml
assert(index <= length(queue))
for i=index:length(queue)-1;
    queue(i) = queue(i+1);
end
queue(length(queue)) = packet(0,0,0,0,0,0);

function num = queueNumElements(queue)
%#eml
num = 0;
for i = 1:length(queue)
    if queue(i).to ~= uint8(0)
        num = num+1;
    end
end    

function packetString = toString(packet) %#eml
eml.extrinsic('sprintf');
packetString = sprintf('%3u: %u->%u :%3u (%.1f) @%.2f', packet.pkgid, packet.from, packet.to, packet.msg, packet.param, packet.time);

== matlab function UserInterface/Link Layer HMI_END.master/Receive Packet ==
  data: packetFrom input; packetMsg input; packetParam input; eventQueueIn input uint8; eventParamQueueIn input double; eventQueue output uint8; eventParamQueue output double; bufferOverflow output boolean
function [eventQueue, eventParamQueue, bufferOverflow] = receivePacket(packetFrom, packetMsg, packetParam, eventQueueIn, eventParamQueueIn)
%#eml
% This function receives packets and adds them to the event queue.
% A packet consists of a source, a message and an optional parameter for 
% the message. Source and message are contained at position 1 and 2 in the 
% eventQueue. Because of the different data type the parameter has his own 
% queue eventParamQueue.

%Constants
SOURCE = 2;
MESSAGE = 1;
BUS_SIZE = numel(packetFrom);
QUEUE_SIZE = 10;

%Init
eventQueue = eventQueueIn;
eventParamQueue = eventParamQueueIn;
bufferOverflow = false;

%New incoming packet
for i = 1:BUS_SIZE
    if packetFrom(i) ~= 0 
        bufferOverflow = true;
        %Add it to the incoming event Queue
        for j = 1:QUEUE_SIZE
            %Search for an empty place
            if eventQueue(j,SOURCE) == 0
                eventQueue(j,SOURCE)    = packetFrom(i);
                eventQueue(j,MESSAGE)   = packetMsg(i);
                eventParamQueue(j)      = packetParam(i);
                bufferOverflow = false;
                break;
            end
        end        
    else
        break;
    end
end

== matlab function UserInterface/Link Layer HMI_END.master/Send Packet ==
  data: busSizeSignal input; eventQueueIn input uint8; eventParamQueueIn input double; packetMsg output; packetParam output; eventQueue output uint8; eventParamQueue output double
function [packetMsg, packetParam, eventQueue, eventParamQueue] = sendPacket(busSizeSignal, eventQueueIn, eventParamQueueIn)
%#eml

% This function creates packets from the event queue. A packet consists
% of a destination, a message and an optional parameter for the message.
% Destination and message are contained at position 1 and 2 in the 
% eventQueue. Because of the different data type the parameter has his own 
% queue eventParamQueue.

%Constants
DESTINATION = 2;
MESSAGE = 1;
QUEUE_SIZE = 10;

busSize = numel(busSizeSignal);

%Init
eventQueue = eventQueueIn;
eventParamQueue = eventParamQueueIn;
packetMsg = zeros(1,busSize,'uint16');
packetParam = zeros(1,busSize,'double');

%There is an event in the queue
for i = 1:busSize   
    if eventQueue(1,DESTINATION) ~= 0 || eventQueue(1,MESSAGE) ~= 0
        %Create packet from the firs entry in the queue
        packetMsg(i)   = uint16(eventQueue(1,MESSAGE));
        packetParam(i) = eventParamQueue(1);
        %Remove the event from the queue
        for j=1:QUEUE_SIZE - 1
            eventQueue(j,DESTINATION)   = eventQueue(j+1,DESTINATION);
            eventQueue(j,MESSAGE)       = eventQueue(j+1,MESSAGE);
            eventParamQueue(j)          = eventParamQueue(j+1);
        end
        %Set last element to zero
        eventQueue(QUEUE_SIZE,DESTINATION)  = 0;
        eventQueue(QUEUE_SIZE,MESSAGE)      = 0;
        eventParamQueue(QUEUE_SIZE)    = 0;
    else
        break;
    end
end
